simulink model "NED_INS_GNSS"  (R2020a)
settings: Solver=FixedStepDiscrete  StartTime=0.0  StopTime=60  FixedStep=0.01  RelTol=1e-3
InitFcn:
  | load('GPS1hz_INS_Car_60s.mat');
undefined symbols (not defined in the file): C_b_n0, h_b0, L_b0, lambda_b0, v_eb_n0
settings Model: Creator=Toranj  LastModifiedBy=Toranj

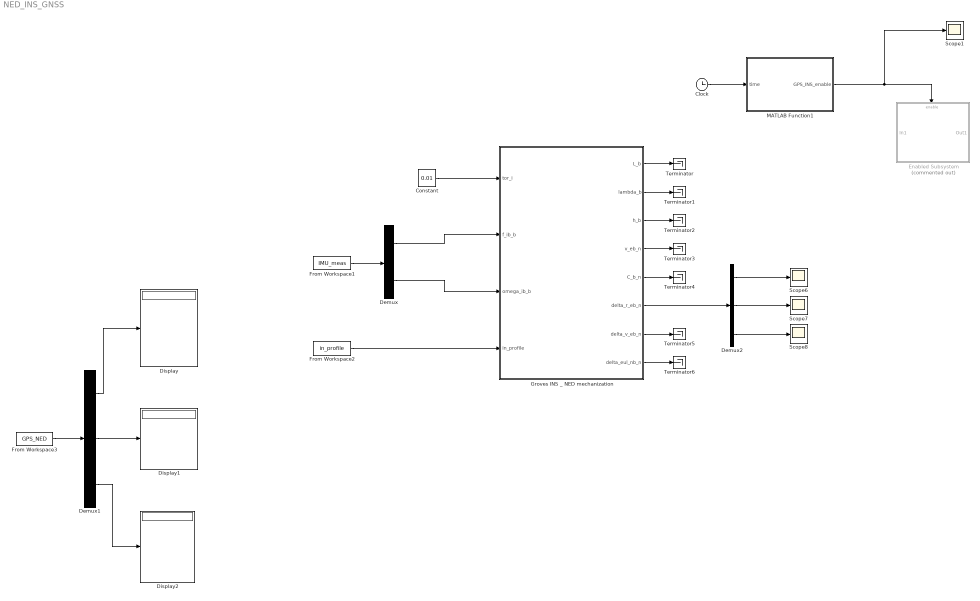
== system NED_INS_GNSS ==
  Clock : Clock
  Constant : Constant  Value=0.01
  Demux : Demux  Outputs=2
  Demux1 : Demux  Outputs=3
  Demux2 : Demux  Outputs=3
  Display : Display
  Display1 : Display
  Display2 : Display
  Enabled Subsystem : Subsystem  Commented=on  TreatAsAtomicUnit=on
  From Workspace1 : FromWorkspace  VariableName=IMU_meas
  From Workspace2 : FromWorkspace  VariableName=in_profile
  From Workspace3 : FromWorkspace  VariableName=GPS_NED
  Groves INS _ NED mechanization : MATLAB Function  TreatAsAtomicUnit=on  mask{old_true_L_b=0.890117918520000, old_true_lambda_b=0, old_true_h_b=10, old_true_v_eb_n=[0;0;0], old_true_C_b_n=eye(3)}
      mask prompts: old_true_L_b "Init_L_b"; old_true_lambda_b "Init_lambda_b"; old_true_h_b "Init_h_b"; old_true_v_eb_n "Init_v_eb_n"; old_true_C_b_n "Init_true_C_b_n"
      mask init:
      | deg_to_rad = 0.01745329252;
      | % rad_to_deg = 1/deg_to_rad;
      | % micro_g_to_meters_per_second_squared = 9.80665E-6;
      | 
      | % Position initialization error (m; N,E,D)
      | initialization_errors.delta_r_eb_n = [4;2;3];
      | % Velocity initialization error (m/s; N,E,D)
      | initialization_errors.delta_v_eb_n = [0.05;-0.05;0.1];
      | % Attitude initialization error (deg, converted to rad; @N,E,D)
      | initialization_errors.delta_eul_nb_n = [-0.05;0.04;1]*deg_to_rad; % rad
      | 
      | [L_b0,lambda_b0,h_b0,v_eb_n0,C_b_n0] =...
      |     Initialize_NED(old_true_L_b,old_true_lambda_b,old_true_h_b,...
      |     old_true_v_eb_n,old_true_C_b_n,initialization_errors);
  MATLAB Function1 : MATLAB Function  TreatAsAtomicUnit=on
  Scope{1,6..8} (4 alike) : Scope
  Terminator{,1..6} (7 alike) : Terminator
  wires:
  From Workspace1/1 -> Demux/1
  Demux/1 -> Groves INS _ NED mechanization/2(f_ib_b)
  Demux/2 -> Groves INS _ NED mechanization/3(omega_ib_b)
  Constant/1 -> Groves INS _ NED mechanization/1(tor_i)
  From Workspace2/1 -> Groves INS _ NED mechanization/4(in_profile)
  Groves INS _ NED mechanization/6(delta_r_eb_n) -> Demux2/1
  Demux2/1 -> Scope6/1
  Demux2/2 -> Scope7/1
  Demux2/3 -> Scope8/1
  Groves INS _ NED mechanization/1(L_b) -> Terminator/1
  Groves INS _ NED mechanization/2(lambda_b) -> Terminator1/1
  Groves INS _ NED mechanization/3(h_b) -> Terminator2/1
  Groves INS _ NED mechanization/4(v_eb_n) -> Terminator3/1
  Groves INS _ NED mechanization/5(C_b_n) -> Terminator4/1
  Groves INS _ NED mechanization/7(delta_v_eb_n) -> Terminator5/1
  Groves INS _ NED mechanization/8(delta_eul_nb_n) -> Terminator6/1
  From Workspace3/1 -> Demux1/1
  Demux1/1 -> Display/1
  Demux1/2 -> Display1/1
  Demux1/3 -> Display2/1
  Clock/1 -> MATLAB Function1/1(time)
  MATLAB Function1/1(GPS_INS_enable) -> Scope1/1, Enabled Subsystem/Enable

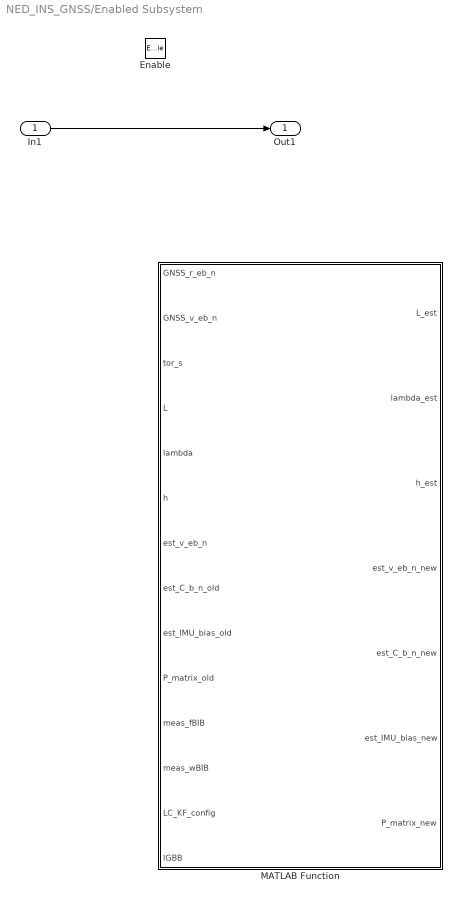
== system NED_INS_GNSS/Enabled Subsystem ==
  In1 : Inport
  Enable : EnablePort
  MATLAB Function : MATLAB Function  TreatAsAtomicUnit=on
  Out1 : Outport
  wires:
  In1/1 -> Out1/1

== matlab function NED_INS_GNSS/Enabled Subsystem/MATLAB Function ==
  data: GNSS_r_eb_n input; L_est output; GNSS_v_eb_n input; tor_s input; L input; lambda input; h input; est_v_eb_n input; est_C_b_n_old input; est_IMU_bias_old input; P_matrix_old input; meas_fBIB input; meas_wBIB input; LC_KF_config input; lGBB input; lambda_est output; h_est output; est_v_eb_n_new output; est_C_b_n_new output; est_IMU_bias_new output; P_matrix_new output
function [L_est,lambda_est,h_est,est_v_eb_n_new,est_C_b_n_new,est_IMU_bias_new,P_matrix_new] =...
    LC_KF_NED(GNSS_r_eb_n,GNSS_v_eb_n,tor_s,L,lambda,h,est_v_eb_n,est_C_b_n_old,est_IMU_bias_old,...
    P_matrix_old,meas_fBIB,meas_wBIB,LC_KF_config,lGBB)

D2R = 0.01745329252;%         convert degree to radian
R2D = 1/D2R;%                 convert radian to degree
Mug2mps2 = 9.80665E-6;%       convert micro-g to meter per second.^2
%% Run the Kalman filter + INS correction
%--------------------------------------------------------------------------
% Inputs:
%   rBEN_GPS        GPS estimated position (m)(@NED)
%   vBEN_GPS        GPS estimated velocity (m/s) (@NED)
%   tao_GPS         propagation interval (s)
%   L               previous latitude (rad)
%   lambda          previous longitude (rad)
%   h               previous height (m)
%   vBEN            prior estimated velocity @ NED frame (m/s)
%   TNB             prior estimated body to NED coordinate transformation matrix
%   IMU_bias_est    prior estimated IMU biases 
%   Cov_est         prior Kalman filter error covariance matrix
%   meas_fBIB       measured specific force of body w.r.t ECI  (m/s^2)
%   meas_wBIB       measured angular rate of body w.r.t ECI    (rad/s)
%   KF_unc          Kalman filter uncertainties
%   lGBB            Lever Arm
%--------------------------------------------------------------------------
% Outputs:
%   L_est           estimated latitude (rad)
%   lambda_est      estimated longitude (rad)
%   h_est           estimated height (m)
%   vBEN_est        estimated velocity @ NED frame (m/s)
%   TNB_est         estimated body to NED coordinate transformation matrix
%   IMU_bias_est    estimated IMU biases
%   Cov_est         estimated Kalman filter error covariance matrix
%==========================================================================
%% Preliminary calculations
%Constant Parameters
omega_ie = 7.292115E-5;   %Earth rotation rate (rad/s)
R0 = 6378137;        %WGS84 Equatorial radius (m)
e = 0.0818191908425; %WGS84 eccentricity

% Copyright 2012, Paul Groves
% License: BSD; see license.txt for details

% Begins

% Skew symmetric matrix of Earth rate
Omega_ie = Skew_symmetric([0,0,omega_ie]);
%--------------------------------------------------------------------------
%Calculate meridian & normal radius of the earth
[R_N,R_E]= Radii_of_curvature(L);
%abbreviation
REh = R_E + h;   RNh = R_N + h; 
vN  = est_v_eb_n(1);   vE = est_v_eb_n(2);   vD = est_v_eb_n(3);
sL  = sin(L);    cL = cos(L);    tL = tan(L);
%Calculate the earth rotation rate @ NED-frame
wNEN = [ vE / (REh);...
        -vN / (RNh);...
        -vE * tL / (REh)];
wEIN = omega_ie * [cL; 0; - sL];    
wNIN = wNEN + wEIN;
%Skew symmetric matrix
WEIN = Skew_symmetric(wEIN);
WNIN = Skew_symmetric(wNIN);
%==========================================================================
%% Determine state transition matrix using ??:
F11 = - WNIN;
F12 = [         0,   -1 / (REh),   0;...
        1 / (RNh),            0,   0;...
                0,   tL / (REh),   0];
%--------------------------------------------------------------------------                      
F13_31 = omega_ie * cL + vE / ((REh) * cL^2);                      
F13 = [ omega_ie * sL,   0,         vE / (REh)^2;...
               0,   0,        -vN / (RNh)^2;...
         F13_31 ,   0,   -vE * tL / (REh)^2];
%--------------------------------------------------------------------------
F21 = -Skew_symmetric(est_C_b_n_old * meas_fBIB);
%--------------------------------------------------------------------------
F22 = [ vD / RNh,    -2 * vE * tL / REh,   vN / RNh;...
               0,   (vN * tL + vD) / REh,  vE / REh;...
               0,                     0,          0];
F22 (2,1) = - F22 (1,2) /2; F22 (3,1) = - 2 * F22 (1,3); F22 (3,2) = - 2 * F22 (2,3);
F22 = F22 -2 * Skew_symmetric(wEIN);
%--------------------------------------------------------------------------
%geocentric radius using B.4:
rSEE = R0 / sqrt(1 - (e * sL)^2) * sqrt(cL^2 + (1 - e^2)^2 * sL^2);
%Calculate surface gravity using the Somigliana model using B.13, B.14:
sL2 = sL^2;
g0 = 9.7803253359 * (1 + 0.001931853 * sL2) / sqrt(1 - e^2 * sL2);
    %-------------------------------------------------------------
F23_1 = [                    - (vE / cL)^2 / REh - 2 * vE * omega_ie * cL;...
         vN * vE/ cL^2 / REh + 2 * vN * omega_ie * cL - 2 * vD * omega_ie * sL;... 
                                                   2 * vE * omega_ie * sL];
F23_3 = [         - (vE / REh)^2 * tL - vN * vD/ RNh^2;...
                     - (vN * vE * tL + vE * vD)/ REh^2;... 
          (vE / REh)^2 + (vN / RNh)^2 - 2 * g0 / rSEE];  
F23 = [ F23_1,   zeros(3,1),   F23_3];   
%--------------------------------------------------------------------------
F32 = [1 / RNh,               0,    0;...
             0,    1 / REh / cL,    0;...
             0,               0,   -1];
%--------------------------------------------------------------------------
F33 = [0, 0, -vN / RNh^2; vE * sL / REh / cL^2, 0, -vE / REh^2 / cL; 0, 0, 0];
%--------------------------------------------------------------------------           
% FN = zeros(15);
% FN(1:3,1:3)   = - WNIN ;
% FN(1:3,4:6)   = F12;
% FN(1:3,7:9)   = F13;
% FN(1:3,13:15) = est_C_b_n_old;
% FN(4:6,1:3)   = F21;
% FN(4:6,4:6)   = F22;
% FN(4:6,7:9)   = F23;
% FN(4:6,10:12) = est_C_b_n_old;
% FN(7:9,4:6)   = F32;
% FN(7:9,7:9)   = F33;
%--------------------------------------------------------------------------
%Continuous to Discrete Model: 
% delta_X'(t)  = FN * X(t)
% delta_X(k+1) = Phi_N * delta_X(k)
% [Phi_matrix,~] = Con2Dis(FN,0,tao_GPS,4);

% 1. Determine transition matrix using (14.50) (first-order approx)
Phi_matrix = eye(15);
Phi_matrix(1:3,1:3) = Phi_matrix(1:3,1:3) + F11 * tor_s;
Phi_matrix(1:3,4:6) = F12 * tor_s;;
Phi_matrix(1:3,7:9) = F13 * tor_s;;
Phi_matrix(1:3,13:15) = est_C_b_n_old * tor_s;

Phi_matrix(4:6,1:3) = F21 * tor_s;
Phi_matrix(4:6,4:6) = Phi_matrix(4:6,4:6) + F22 * tor_s;
Phi_matrix(4:6,7:9) = F23 * tor_s;
Phi_matrix(4:6,10:12) = est_C_b_n_old * tor_s;

Phi_matrix(7:9,4:6) = F32 * tor_s;
Phi_matrix(7:9,7:9) = Phi_matrix(7:9,7:9) + F33 * tor_s;

% Phi_matrix(1:3,1:3) = Phi_matrix(1:3,1:3) - Omega_ie * tor_s;
% Phi_matrix(1:3,13:15) = est_C_b_e_old * tor_s;
% Phi_matrix(4:6,1:3) = -tor_s * Skew_symmetric(est_C_b_e_old * meas_f_ib_b);
% Phi_matrix(4:6,4:6) = Phi_matrix(4:6,4:6) - 2 * Omega_ie * tor_s;
% geocentric_radius = R_0 / sqrt(1 - (e * sin(est_L_b_old))^2) *...
%     sqrt(cos(est_L_b_old)^2 + (1 - e^2)^2 * sin(est_L_b_old)^2); % from (2.137)
% Phi_matrix(4:6,7:9) = -tor_s * 2 * Gravity_ECEF(est_r_eb_e_old) /...
%     geocentric_radius * est_r_eb_e_old' / sqrt (est_r_eb_e_old' *...
%     est_r_eb_e_old);
% Phi_matrix(4:6,10:12) = est_C_b_e_old * tor_s;
% Phi_matrix(7:9,4:6) = eye(3) * tor_s;
%==========================================================================
%% Determine exact system noise covariance matrix using 1.44, 1.45:
tao_INS = 0.01;
    %init_ba_sd: Initial accel. bias uncertainty (m/s^2)
    init_ba_sd = 1000 * Mug2mps2;
    %accel_VRW: Accelerometer noise PSD (m^2 s^-3)
    accel_VRW = (1100 * Mug2mps2) ^ 2 * tao_INS;
    %accel_bias_PSD: Accelerometer bias random walk PSD (m^2 s^-5)
    accel_bias_PSD = 1.0E-5;
    %init_bg_sd: Initial gyro. bias uncertainty (rad/s)
    init_bg_sd = 20 * D2R / 3600;
    %gyro_ARW: Gyro noise PSD (rad^2/s)
    gyro_ARW = (1.1 * D2R / 60)^ 2 * tao_INS;
    %gyro_bias_PSD: Gyro bias random walk PSD (rad^2 s^-3)
    gyro_bias_PSD = 4.0E-11;
%-------------------------------------------------------------------------- 
%% IMU noise uncertainty
KF_unc.noise_IMU = [accel_VRW; gyro_ARW;  accel_bias_PSD;  gyro_bias_PSD;];

S_a  = KF_unc.noise_IMU (1);
S_g  = KF_unc.noise_IMU (2);
Sp_a = KF_unc.noise_IMU (3);
Sp_g = KF_unc.noise_IMU (4);
%Cartesian-to-curvilinear position change transformation matrix (p = T_prn * r_n)
T_prn = F32;
%--------------------------------------------------------------------------
Q11 = eye(3) * (S_g * tor_s + Sp_g * tor_s^3 / 3);
Q15 = Sp_g*tor_s^2*est_C_b_n_old / 2;
Q21 = (S_g*tor_s^2 / 2 + Sp_g*tor_s^4 / 4) * F21;
Q22 = (S_a*tor_s + Sp_a*tor_s^3/3)*eye(3) + (S_g*tor_s^3/3 + Sp_g*tor_s^5/5)*(F21*F21');
Q24 = Sp_a*tor_s^2*est_C_b_n_old / 2;
Q25 = Sp_g*tor_s^3*F21*est_C_b_n_old / 3;
Q31 = (S_g*tor_s^3 / 3 + Sp_g*tor_s^5 / 5) * T_prn * F21;
Q32 = (S_a*tor_s^2/2 + Sp_a*tor_s^4/4) * T_prn + (S_g*tor_s^4/4 + Sp_g*tor_s^6/6)*(T_prn*(F21*F21'));
Q33 = (S_a*tor_s^3/3 + Sp_a*tor_s^5/5)*T_prn*T_prn + (S_g*tor_s^5/5 + Sp_g*tor_s^7/7)*T_prn*(F21*F21')*T_prn;
Q34 = Sp_a*tor_s^3*T_prn*est_C_b_n_old/3;
Q35 = Sp_g*tor_s^4*T_prn*F21*est_C_b_n_old/4;
Q44 = Sp_a*tor_s*eye(3);
Q55 = Sp_g*tor_s*eye(3);
Q_prime_matrix = [Q11        Q21'    Q31'    zeros(3)    Q15;
       Q21        Q22     Q32'    Q24         Q25;
       Q31        Q32     Q33     Q34         Q35;
       zeros(3)   Q24'    Q34'    Q44         zeros(3);
       Q15'       Q25'    Q35'    zeros(3)    Q55;];
%==========================================================================
%% Propagation 
% 3. Propagate state estimates using (3.14) noting that all states are zero 
% due to closed-loop correction.
x_est_propagated(1:15,1) = 0;
%--------------------------------------------------------------------------
% 4. Propagate state estimation error covariance matrix using (3.46)
P_matrix_propagated = Phi_matrix * (P_matrix_old + 0.5 * Q_prime_matrix) *...
    Phi_matrix' + 0.5 * Q_prime_matrix;
%==========================================================================
% MEASUREMENT UPDATE PHASE     

%rescale the latitude and longitude components
S_Ll = 1E3;
Sp = diag ([S_Ll, S_Ll, 1]);
% 5. Set-up measurement matrix using (14.115) 
H_matrix = zeros(6,15);
H_matrix(1:3,1:3)   =  Sp * (T_prn * Skew_symmetric(est_C_b_n_old * lGBB));
H_matrix(1:3,7:9)   = -Sp;
H_matrix(4:6,1:3)   = Skew_symmetric(est_C_b_n_old * cross(meas_wBIB,lGBB) - WEIN * est_C_b_n_old * lGBB);
H_matrix(4:6,4:6)   = -eye(3);
H_matrix(4:6,13:15) = est_C_b_n_old * Skew_symmetric(lGBB);

p = [L; lambda; h];
%Formulate measurement innovations using 1.53:
delta_z(1:3,1) = Sp * (GNSS_r_eb_n - p - T_prn * est_C_b_n_old * lGBB);
delta_z(4:6,1) = GNSS_v_eb_n - est_v_eb_n - est_C_b_n_old * cross(meas_wBIB,lGBB)+ WEIN * est_C_b_n_old * lGBB;
%--------------------------------------------------------------------------
%Set-up measurement matrix using 1.50, 1.52:
% H = zeros(6,15);
% H(1:3,1:3)   =  Sp * (T_prn * Skew_symmetric(est_C_b_n_old * lGBB));
% H(1:3,7:9)   = -Sp;
% H(4:6,1:3)   = Skew_symmetric(est_C_b_n_old * cross(meas_wBIB,lGBB) - WEIN * est_C_b_n_old * lGBB);
% H(4:6,4:6)   = -eye(3);
% H(4:6,13:15) = est_C_b_n_old * Skew_symmetric(lGBB);
%--------------------------------------------------------------------------
%Set-up measurement noise covariance matrix 
% R_matrix = KF_unc.Cov_meas;
% 6. Set-up measurement noise covariance matrix assuming all components of
% GNSS position and velocity are independent and have equal variance.
R_matrix(1:3,1:3) = eye(3) * LC_KF_config.pos_meas_SD^2;
R_matrix(1:3,4:6) = zeros(3);
R_matrix(4:6,1:3) = zeros(3);
R_matrix(4:6,4:6) = eye(3) * LC_KF_config.vel_meas_SD^2;
%==========================================================================
%% Estimation
% 7. Calculate Kalman gain using (3.21)
K_matrix = P_matrix_propagated * H_matrix' /(H_matrix *P_matrix_propagated * H_matrix' + R_matrix);
%--------------------------------------------------------------------------
% 9. Update state estimates using (3.24)
x_est_new = x_est_propagated + K_matrix * delta_z;
%--------------------------------------------------------------------------
% 10. Update state estimation error covariance matrix using (3.25)
P_matrix_new = (eye(15) - K_matrix * H_matrix) * P_matrix_propagated;
%==========================================================================
%% CLOSED-LOOP CORRECTION
% Correct attitude 
est_C_b_n_new = (eye(3) - Skew_symmetric(x_est_new(1:3))) * est_C_b_n_old;
%Orthonormalization
% est_C_b_n_new = OrthoNorm(est_C_b_n_new);
%--------------------------------------------------------------------------
%Correct velocity
est_v_eb_n_new = est_v_eb_n - x_est_new(4:6);
%--------------------------------------------------------------------------
%Correct position
L_est      = p(1) - x_est_new(7);
lambda_est = p(2) - x_est_new(8);
h_est      = p(3) - x_est_new(9);
%--------------------------------------------------------------------------
% Update IMU bias estimates
est_IMU_bias_new = est_IMU_bias_old + x_est_new(10:15);
%==========================================================================
end

== matlab function NED_INS_GNSS/Groves INS _ NED mechanization ==
  data: tor_i input; L_b output; f_ib_b input; omega_ib_b input; in_profile input; lambda_b output; h_b output; v_eb_n output; C_b_n output; L_b0 parameter; lambda_b0 parameter; h_b0 parameter; v_eb_n0 parameter; C_b_n0 parameter; delta_r_eb_n output; delta_v_eb_n output; delta_eul_nb_n output
% function [L_b,lambda_b,h_b,v_eb_n,C_b_n] = Nav_equations_NED(tor_i,...
%         old_L_b,old_lambda_b,old_h_b,old_v_eb_n,old_C_b_n,f_ib_b,omega_ib_b)
function [L_b,lambda_b,h_b,v_eb_n,C_b_n,...
    delta_r_eb_n,delta_v_eb_n,delta_eul_nb_n] = Nav_equations_NED(tor_i,...
    f_ib_b,omega_ib_b,in_profile, L_b0, lambda_b0, h_b0, v_eb_n0, C_b_n0)
%Nav_equations_NED - Runs precision local-navigation-frame inertial
%navigation equations (Note: only the attitude update and specific force
%frame transformation phases are precise.)
%
% Software for use with "Principles of GNSS, Inertial, and Multisensor
% Integrated Navigation Systems," Second Edition.
%
% This function created 1/4/2012 by Paul Groves
%
% Inputs:
%   tor_i         time interval between epochs (s)
%   old_L_b       previous latitude (rad)
%   old_lambda_b  previous longitude (rad)
%   old_h_b       previous height (m)
%   old_C_b_n     previous body-to-NED coordinate transformation matrix
%   old_v_eb_n    previous velocity of body frame w.r.t. ECEF frame, resolved
%                 along north, east, and down (m/s)
%   f_ib_b        specific force of body frame w.r.t. ECEF frame, resolved
%                 along body-frame axes, averaged over time interval (m/s^2)
%   omega_ib_b    angular rate of body frame w.r.t. ECEF frame, resolved
%                 about body-frame axes, averaged over time interval (rad/s)
% Outputs:
%   L_b           latitude (rad)
%   lambda_b      longitude (rad)
%   h_b           height (m)
%   v_eb_n        velocity of body frame w.r.t. ECEF frame, resolved along
%                 north, east, and down (m/s)
%   C_b_n         body-to-NED coordinate transformation matrix

% Copyright 2012, Paul Groves
% License: BSD; see license.txt for details

% parameters
omega_ie = 7.292115E-5;  % Earth rotation rate (rad/s)

% Begins
persistent old_L_b old_lambda_b old_h_b old_v_eb_n old_C_b_n;
if isempty(old_L_b)
    old_L_b = L_b0;
    old_lambda_b = lambda_b0;
    old_h_b = h_b0;
    old_v_eb_n = v_eb_n0;
    old_C_b_n = C_b_n0;
end
% PRELIMINARIES
% Calculate attitude increment, magnitude, and skew-symmetric matrix
alpha_ib_b = omega_ib_b * tor_i;
mag_alpha = sqrt(alpha_ib_b' * alpha_ib_b);
Alpha_ib_b = Skew_symmetric(alpha_ib_b);

% From (2.123) , determine the angular rate of the ECEF frame
% w.r.t the ECI frame, resolved about NED
omega_ie_n = omega_ie * [cos(old_L_b); 0; - sin(old_L_b)];

% From (5.44), determine the angular rate of the NED frame
% w.r.t the ECEF frame, resolved about NED
[old_R_N,old_R_E] = Radii_of_curvature(old_L_b);
old_omega_en_n = [old_v_eb_n(2) / (old_R_E + old_h_b);...
    -old_v_eb_n(1) / (old_R_N + old_h_b);...
    -old_v_eb_n(2) * tan(old_L_b) / (old_R_E + old_h_b)];

% SPECIFIC FORCE FRAME TRANSFORMATION
% Calculate the average body-to-ECEF-frame coordinate transformation
% matrix over the update interval using (5.84) and (5.86)
if mag_alpha>1.E-8
    ave_C_b_n = old_C_b_n * (eye(3) + (1 - cos(mag_alpha)) / mag_alpha^2 ...
        * Alpha_ib_b + (1 - sin(mag_alpha) / mag_alpha) / mag_alpha^2 ...
        * Alpha_ib_b * Alpha_ib_b) -...
        0.5 * Skew_symmetric(old_omega_en_n + omega_ie_n) * old_C_b_n;
else
    ave_C_b_n = old_C_b_n -...
        0.5 * Skew_symmetric(old_omega_en_n + omega_ie_n) * old_C_b_n;
end %if mag_alpha

% Transform specific force to ECEF-frame resolving axes using (5.86)
f_ib_n = ave_C_b_n * f_ib_b;

% UPDATE VELOCITY
% From (5.54),
v_eb_n = old_v_eb_n + tor_i * (f_ib_n + Gravity_NED(old_L_b,old_h_b) -...
    Skew_symmetric(old_omega_en_n + 2 * omega_ie_n) * old_v_eb_n);

% UPDATE CURVILINEAR POSITION
% Update height using (5.56)
h_b = old_h_b - 0.5 * tor_i * (old_v_eb_n(3) + v_eb_n(3));

% Update latitude using (5.56)
L_b = old_L_b + 0.5 * tor_i * (old_v_eb_n(1) / (old_R_N + old_h_b) +...
    v_eb_n(1) / (old_R_N + h_b));

% Calculate meridian and transverse radii of curvature
[R_N,R_E]= Radii_of_curvature(L_b);

% Update longitude using (5.56)
lambda_b = old_lambda_b + 0.5 * tor_i * (old_v_eb_n(2) / ((old_R_E +...
    old_h_b) * cos(old_L_b)) + v_eb_n(2) / ((R_E + h_b) * cos(L_b)));

% ATTITUDE UPDATE
% From (5.44), determine the angular rate of the NED frame
% w.r.t the ECEF frame, resolved about NED
omega_en_n = [v_eb_n(2) / (R_E + h_b);...
    -v_eb_n(1) / (R_N + h_b);...
    -v_eb_n(2) * tan(L_b) / (R_E + h_b)];

% Obtain coordinate transformation matrix from the new attitude w.r.t. an
% inertial frame to the old using Rodrigues' formula, (5.73)
if mag_alpha>1.E-8
    C_new_old = eye(3) + sin(mag_alpha) / mag_alpha * Alpha_ib_b +...
        (1 - cos(mag_alpha)) / mag_alpha^2 * Alpha_ib_b * Alpha_ib_b;
else
    C_new_old = eye(3) + Alpha_ib_b;
end %if mag_alpha

% Update attitude using (5.77)
C_b_n = (eye(3) - Skew_symmetric(omega_ie_n + 0.5 * omega_en_n + 0.5 *...
    old_omega_en_n)  * tor_i) * old_C_b_n * C_new_old;



true_L_b = in_profile(1);
true_lambda_b = in_profile(2);
true_h_b = in_profile(3);
true_v_eb_n = in_profile(4:6);
true_eul_nb = in_profile(7:9);
true_C_b_n = Euler_to_CTM(true_eul_nb)';
[delta_r_eb_n,delta_v_eb_n,delta_eul_nb_n] = Calculate_errors_NED(...
    L_b,lambda_b,h_b,v_eb_n,C_b_n,true_L_b,...
    true_lambda_b,true_h_b,true_v_eb_n,true_C_b_n);

old_L_b = L_b;
old_lambda_b = lambda_b;
old_h_b = h_b;
old_v_eb_n = v_eb_n;
old_C_b_n = C_b_n;
% Ends

== matlab function NED_INS_GNSS/MATLAB Function1 ==
  data: time input; GPS_INS_enable output
function GPS_INS_enable = fcn(time)

persistent GPS_update_time

if isempty(GPS_update_time)
    GPS_update_time=0;
end

    if (time - GPS_update_time) >= 1 % Time update interval
        GPS_INS_enable = 1;
        GPS_update_time = time;
    else
        GPS_INS_enable = 0;
    end
    
end
